simulink model "Task29"  (R2025a)
settings: Solver=VariableStepAuto  StartTime=0.0  StopTime=10.0  RelTol=1e-3
settings Model: Creator=LOQ  LastModifiedBy=LOQ

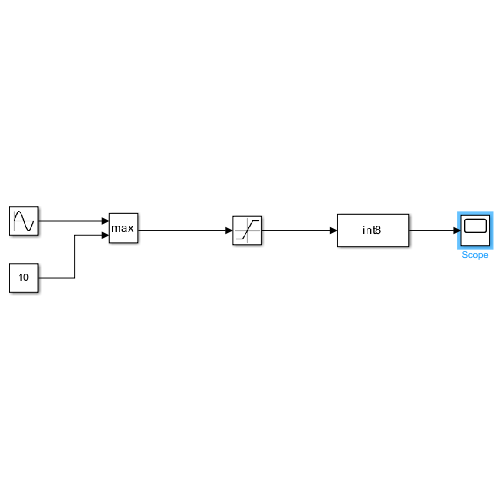
[thumbnail: Simulink's stored preview of the top-level diagram]
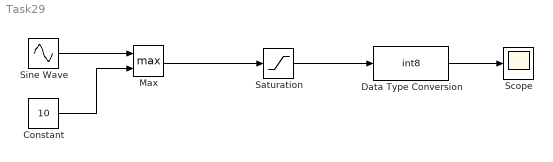
== system Task29 ==
  Constant : Constant  Value=10
  Data Type Conversion : DataTypeConversion  OutDataTypeStr=int8  SaturateOnIntegerOverflow=off  RndMeth=Floor
  Max : MinMax  Function=max  Inputs=2
  Saturation : Saturate  UpperLimit=90  LowerLimit=0
  Scope : Scope
      settings: ActiveDisplayYMinimum=1.7763568394002505E-15  ActiveDisplayYMaximum=100
  Sine Wave : Sin  Amplitude=100  SampleTime=0
  wires:
  Constant/1 -> Max/2
  Sine Wave/1 -> Max/1
  Max/1 -> Saturation/1
  Saturation/1 -> Data Type Conversion/1
  Data Type Conversion/1 -> Scope/1
